simulink model "PLANTA_COMPLETA"  (R2024b)
settings: Solver=FixedStepAuto  StartTime=0.0  StopTime=inf  FixedStep=0.001  MaxStep=0.0005  RelTol=1e-4
undefined symbols (not defined in the file): A_hm, A_tm, at_breakpoints, at_max, b_ha, B_hm, b_ta, B_tm, bcx, bcy, bhd, bhEb, bhm, bt, btd, btm, btw, bwu, C_hm, C_tm, D_hm, D_tm, DiscIntNeverNeededParam, dl_h_ini, dx_l_ini, dx_t_ini, dx_td_ini, dxt_max, dy_l_ini, F01_a_t_max, F01_Ts1, F02_a_h_max, F02_Ts1, F03_a_h_max, F03_a_t_max, F03_dxt_max, F03_Ts1, Fhw_min, g, Hc, ih, it, Jhd_hEb, Jhm_hb, Jtd, Jtm_tb, K_hsa, K_hsia, K_tsa, K_tsia, Kcy, Kd_table, Ke_tita, Ke_w, kp_pos, Kp_table, kp_w, Ktw, kwu, l_breakpoints ... (+30)
libraries: simulink x13, spsEdgeDetectorLib x5, simulink_extras x2, dspsigops x2, vrlib x1, dspstat3 x1
(part 1 of 5)
settings Model: Creator=ribei  LastModifiedBy=juani
settings SolverCC: ZeroCrossAlgorithm=Adaptive  AutoInsertRateTranBlk=on
settings DebuggingCC: IgnoredZcDiagnostic=none  UnderSpecifiedDimensionMsg=warning

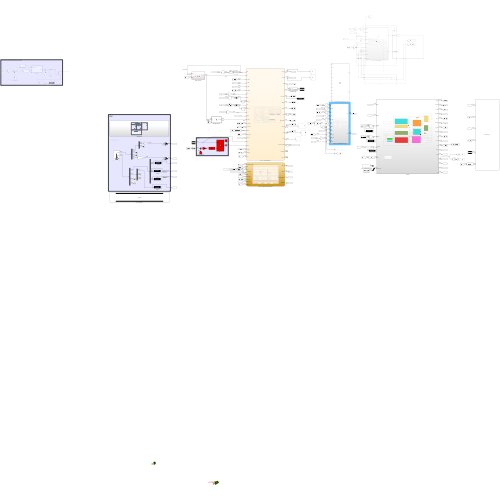
[thumbnail: Simulink's stored preview of the top-level diagram]
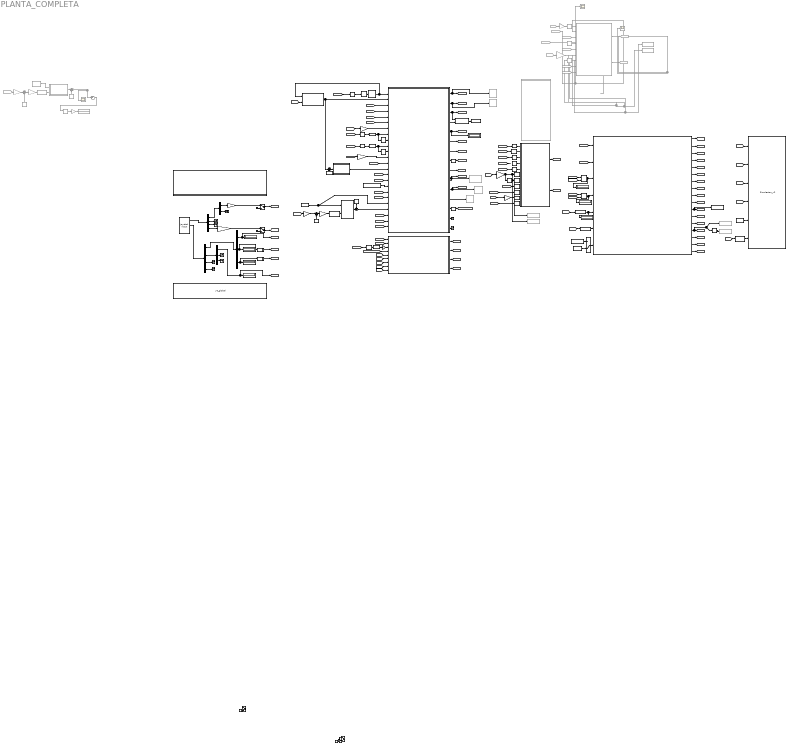
== system PLANTA_COMPLETA ==
  note: SOLO PARA PROBAR ESTIMADOR DE MASA
  note: HMI
  note: LIDAR
  note: CONTROL
  AND : Logic  IconShape=distinctive  AllPortsSameDT=off  OutDataTypeStr=boolean
  AND1 : Logic  IconShape=distinctive  AllPortsSameDT=off  OutDataTypeStr=boolean
  Actualizar perfil : Subsystem
  Ajuste referencia : Constant  Value=30
  Ajuste referencia1 : Constant  Commented=on  Value=30
  Boton A : Display
  Boton B : Display
  Boton X : Display
  Boton Y : Display
  Calculo : MATLAB Function  Commented=on  TreatAsAtomicUnit=on
  Cast : DataTypeConversion  OutDataTypeStr=boolean  SaturateOnIntegerOverflow=off  RndMeth=Floor
  Cast To Boolean : DataTypeConversion  OutDataTypeStr=boolean  SaturateOnIntegerOverflow=off  RndMeth=Floor
  Cast1 : DataTypeConversion  OutDataTypeStr=boolean  SaturateOnIntegerOverflow=off  RndMeth=Floor
  Constant : Constant
  Constant{1..2,18..19,28} (5 alike) : Constant  Value=0  SampleTime=T_s1
  Constant15 : Constant  Value=Yt0
  Constant3 : Constant  Commented=on  Value=Ms
  Constant4 : Constant  Value=30.7948720557058
  Constant5 : Constant  Commented=on
  Constant9 : Constant  Value=Ms
  DASHBOARD : Subsystem
  Data Store Read1 : DataStoreRead  DataStoreName=y0_global  IndexOptions=Index vector (dialog)  Indices=1  OutputSizes=1
  Data Store Read2 : DataStoreRead  DataStoreName=y0_global  IndexOptions=Index vector (dialog)  Indices=1  OutputSizes=1
  Data Store Write : DataStoreWrite  DataStoreName=y0_global  IndexOptions=Index vector (dialog)  Indices=1  OutputSizes=1
  Data Type Conversion : DataTypeConversion  OutDataTypeStr=int32  RndMeth=Ceiling  SaturateOnIntegerOverflow=off
  Data Type Conversion1 : DataTypeConversion  Commented=on  OutDataTypeStr=int32  RndMeth=Ceiling  SaturateOnIntegerOverflow=off
  Delay1 : Delay  DelayLength=1  InputProcessing=Columns as channels (frame based)  SampleTime=T_s1
  Delay2 : Delay  DelayLength=1  InputProcessing=Columns as channels (frame based)  SampleTime=T_s1
  Demux : Demux
  Demux1 : Demux  Outputs=2
  Demux2 : Demux
  Demux3 : Demux  Outputs=3
  Demux4 : Demux  Outputs=3
  Derivative : Derivative  Commented=on
  Derivative1 : Derivative  Commented=on
  Derivative2 : Derivative
  Derivative3 : Derivative
  Discrete Derivative : simulink/Discrete/Discrete Derivative  gainval=1.0  ICPrevScaledInput=0.0  OutMin=[]  OutMax=[]  OutDataType=fixdt(1, 16)  OutScaling=2^-10  DoSatur=off
  Discrete Derivative1 : simulink/Discrete/Discrete Derivative  gainval=1.0  ICPrevScaledInput=0.0  OutMin=[]  OutMax=[]  OutDataType=fixdt(1, 16)  OutScaling=2^-10  DoSatur=off
  Discrete Derivative2 : simulink/Discrete/Discrete Derivative  gainval=1.0  ICPrevScaledInput=0.0  OutMin=[]  OutMax=[]  OutDataType=fixdt(1, 16)  OutScaling=2^-10  DoSatur=off
  Display{,2..4} (4 alike) : Display
  Display1 : Display  Commented=on
  Divide : Product  Commented=on  Inputs=*/
  Enclavamiento : Stateflow chart  TreatAsAtomicUnit=on
  Enclavamiento1 : Stateflow chart  TreatAsAtomicUnit=on
  From1 : From  Commented=on  GotoTag=tita_l
  From11 : From  Commented=on  GotoTag=dxt_ref
  From15 : From  Commented=on  GotoTag=Ml_estimada
  From2 : From  Commented=on  GotoTag=tita_tm
  From21 : From  Commented=on  GotoTag=bal_control
  From22 : From  Commented=on  GotoTag=ddxt_ref
  From3 : From  Commented=on  GotoTag=tita_hm
  From44 : From  Commented=on  GotoTag=dlh_ref
  From5 : From  Commented=on  GotoTag=tita_tm
  Gain : Gain  Gain=1/Wc
  Gain1 : Gain  Commented=on  Gain=rtd/it
  Gain12 : Gain  Gain=rtd/it
  Gain13 : Gain  Gain=-rhd/(ih*2)
  Gain2 : Gain  Commented=on  Gain=-rhd/(ih*2)
  Gain3 : Gain  Gain=rtd/it
  Gain4 : Gain  Gain=rtd/it
  Gain5 : Gain  Gain=-rhd/(ih*2)
  Gain6 : Gain  Commented=on  Gain=1/Wc
  Gain7 : Gain  Commented=on  Gain=rtd/it
  Gain8 : Gain  Gain=rhd/(-2*ih)
  Gain9 : Gain  Commented=on  Gain=100
  Goto10 : Goto  Commented=on  GotoTag=T_tm
  Goto11 : Goto  Commented=on  GotoTag=T_hm
  Joystick Input : vrlib/Joystick Input  joyid=1  adjustports=on  forcefeed=off
  Level-2 MATLAB S-Function : M-S-Function  FunctionName=Simulacion_v2  Parameters=2.438, 2.591, 1.500, 0.850, 0.750, 7.500, 2.100, 2.500, 'black', 'black', '#E99000', 5.000
  Manual Switch{1..4,11} (5 alike) : ManualSwitch
  Manual Switch5 : ManualSwitch  CurrentSetting=0
  Masa contenedor : Subsystem
  Memory1 : Memory  InheritSampleTime=on
  Memory2 : Memory  InheritSampleTime=on
  Moving Average : dspstat3/Moving Average  Method=Sliding window  ForgettingFactorPort=off  SpecifyWindowLength=on  WindowLength=40  OverlapLength=0  AllowArbitraryInputLength=off  ForgettingFactor=0.9  SimulateUsing=Interpreted execution
  Multiply : Gain  Gain=vt_max
  Multiply1 : Gain  Gain=vh_max_sc
  Nivel 0 - Seguridad o Proteccion : Stateflow chart  TreatAsAtomicUnit=on  SystemSampleTime=T_s0
      settings: PortSchema="{\"entries\":[{\"content\":{\"sides\":[{\"content\":{\"connectorIds\":[\"In6\",\"In9\",\"In8\",\"In7\",\"In1\",\"In2\",\"In3\",\"In5\",\"In4\"]},\"type\":\"ConnectorPlacement.EquallySpacedRectSide\",\"uuid\":\"92abb5b4-7f8d-4d16-9e1c-3f1528aec02e\"},{\"content\":{\"connectorIds\":[\"Out2\",\"Out1\",\"Out3\",\"Out4\"],\"side\":\"RIGHT\"},\"type\":\"ConnectorPlacement.EquallySpacedRectSide\",\"uuid\":\"fdfc4918-925b-4492-9924-9f3ed7c6f0ea\"},{\"content\":{\"side\":\"TOP\"},\"type\":\"ConnectorPlacement.EquallySpacedRectSide\",\"uuid\":\"6cd2c614-9727-439b-b51b-96ebe361e1e6\"},{\"content\":{\"side\":\"BOTTOM\"},\"type\":\"ConnectorPlacement.EquallySpacedRectSide\",\"uuid\":\"c327f02f-ffd6-4494-8eea-bb6a75c04a8c\"}]},\"type\":\"ConnectorPlacement.EquallySpacedConnector\",\"uuid\":\"17c891de-27fd-4863-a62e-79c0c94ffbc9\"}],\"packageUris\":[\"http://schema.mathworks.com/mf0/Connector/R2020b\"],\"version\":\"1.0\"}"
  Nivel 1 - Control Supervisor : Stateflow chart  TreatAsAtomicUnit=on  SystemSampleTime=T_s1
  Nivel 2 - Control Regulatorio : Subsystem  Commented=on
  Nivel 2 - Control Regulatorio + Obs : Subsystem
  Nivel 2: Control Regulatorio1 : MATLAB Function  Commented=on  TreatAsAtomicUnit=on  SystemSampleTime=T_s2
  PLANTA : Subsystem
  Perfil de obstaculos : DataStoreMemory  DataStoreName=y0_global  WriteAfterWriteMsg=warning  InitialValue=y0  ShowAdditionalParam=off  OutDataTypeStr=double
  Scope1 : Scope  Commented=on  NumInputPorts=2
  Scope4 : Scope  Commented=on
  Scope5 : Scope  Commented=on
  Sum : Sum  Inputs=|++
  Sum1 : Sum  Inputs=|++
  Sum2 : Sum  Inputs=+-|
  Sum3 : Sum  Commented=on  Inputs=|++
  Sum4 : Sum  Commented=on  Inputs=|++
  Sum5 : Sum  Commented=on  Inputs=-|+||
  Tapped Delay : simulink/Discrete/Tapped Delay  vinit=0.0  samptime=T_s1  NumDelays=40  DelayOrder=Oldest  includeCurrent=off
  Terminator{,1..8} (9 alike) : Terminator
  To Workspace : ToWorkspace  Commented=on  VariableName=xt_ref  SaveFormat=Timeseries  SampleTime=-1
      settings: Save2DSignal=2-D array (concatenate along first dimension)
  To Workspace1 : ToWorkspace  Commented=on  VariableName=ddxt_ref  SaveFormat=Timeseries  SampleTime=-1
      settings: Save2DSignal=2-D array (concatenate along first dimension)
  To Workspace10 : ToWorkspace  Commented=on  VariableName=l_h_real  SaveFormat=Timeseries  SampleTime=-1
      settings: Save2DSignal=2-D array (concatenate along first dimension)
  To Workspace11 : ToWorkspace  Commented=on  VariableName=dl_h_real  SaveFormat=Timeseries  SampleTime=-1
      settings: Save2DSignal=2-D array (concatenate along first dimension)
  To Workspace2 : ToWorkspace  Commented=on  VariableName=dxt_ref  SaveFormat=Timeseries  SampleTime=-1
      settings: Save2DSignal=2-D array (concatenate along first dimension)
  To Workspace3 : ToWorkspace  Commented=on  VariableName=dlh_ref  SaveFormat=Timeseries  SampleTime=-1
      settings: Save2DSignal=2-D array (concatenate along first dimension)
  To Workspace4 : ToWorkspace  Commented=on  VariableName=lh_ref  SaveFormat=Timeseries  SampleTime=-1
      settings: Save2DSignal=2-D array (concatenate along first dimension)
  To Workspace5 : ToWorkspace  Commented=on  VariableName=x_t_real  SaveFormat=Timeseries  SampleTime=-1
      settings: Save2DSignal=2-D array (concatenate along first dimension)
  To Workspace6 : ToWorkspace  Commented=on  VariableName=l_h_real  SaveFormat=Timeseries  SampleTime=-1
      settings: Save2DSignal=2-D array (concatenate along first dimension)
  To Workspace7 : ToWorkspace  Commented=on  VariableName=dl_h_real  SaveFormat=Timeseries  SampleTime=-1
      settings: Save2DSignal=2-D array (concatenate along first dimension)
  To Workspace8 : ToWorkspace  VariableName=tita_real  SaveFormat=Timeseries  SampleTime=-1
      settings: Save2DSignal=2-D array (concatenate along first dimension)
  To Workspace9 : ToWorkspace  Commented=on  VariableName=dx_t_real  SaveFormat=Timeseries  SampleTime=-1
      settings: Save2DSignal=2-D array (concatenate along first dimension)
  Vector de masas : FromWorkspace  VariableName=Mc_Xvect
  Vector de masas sobrecarga : FromWorkspace  VariableName=Mc_Xvect_sobrecarga
  Vector de masas3 : FromWorkspace  Commented=on  VariableName=Mc_Xvect
  Velocidad max izaje : MATLAB Function  TreatAsAtomicUnit=on
  Zero-Order Hold : ZeroOrderHold  SampleTime=T_s1
  Zero-Order Hold1 : ZeroOrderHold  SampleTime=T_s1
  Zero-Order Hold{4..13} (10 alike) : ZeroOrderHold  SampleTime=T_s2
  Zero-Order Hold2 : ZeroOrderHold  SampleTime=T_s1
  Zero-Order Hold3 : ZeroOrderHold  SampleTime=T_s0
  sensor : MATLAB Function  TreatAsAtomicUnit=on
  wires:
  AND/1 -> Display/1, PLANTA/3(BRK_t)
  AND1/1 -> Display3/1, PLANTA/4(BRK_h)
  PLANTA/12(tita_tm) -> [tita_tm]
  PLANTA/13(tita_hm) -> [tita_hm]
  PLANTA/14(x_t) -> Derivative2/1, To Workspace5/1, [x_t]
  PLANTA/15(x_l) -> [x_l]
  PLANTA/16(y_l) -> [y_l]
  Data Store Read2/1 -> Level-2 MATLAB S-Function/5
  [tita_l] -> Level-2 MATLAB S-Function/4
  Gain2/1 -> Nivel 2 - Control Regulatorio/6(l_h), To Workspace10/1, Derivative1/1
  From3/1 -> Gain2/1
  From15/1 -> Nivel 2 - Control Regulatorio/3(m_l)
  Nivel 2 - Control Regulatorio/1(T_tm) -> Scope4/1, Goto10/1
  From2/1 -> Gain1/1  "signal"
  Gain1/1 -> Derivative/1
  Masa contenedor/1(Mc_X) -> Nivel 1 - Control Supervisor/2(Ml), Sum1/1  "signal"
  [FC_SUP] -> Nivel 1 - Control Supervisor/3(FC_SUP)  "signal"
  [FC_INF] -> Nivel 1 - Control Supervisor/4(FC_INF)  "signal"
  [FC_IZQ] -> Nivel 1 - Control Supervisor/5(FC_IZQ)  "signal"
  [FC_DER] -> Nivel 1 - Control Supervisor/6(FC_DER)  "signal"
  Gain3/1 -> Nivel 1 - Control Supervisor/7(xtd)  "signal"
  [tita_hm] -> Zero-Order Hold/1  "signal"
  [tita_tm] -> Zero-Order Hold1/1  "signal"
  Gain5/1 -> Nivel 1 - Control Supervisor/12(lh)  "signal"
  [falla_E] -> Nivel 1 - Control Supervisor/13(falla_E)
  Demux4/1 -> [Boton_A], Boton A/1  "signal"
  Demux4/2 -> Enclavamiento1/1(input), Boton B/1  "signal"
  Constant4/1 -> Nivel 1 - Control Supervisor/17(destino)  "signal"
  Nivel 1 - Control Supervisor/3(TLK) -> [TLK], Actualizar perfil/1(TLK)
  Nivel 1 - Control Supervisor/7(BRK_t) -> [BRK_t_N1]
  Nivel 1 - Control Supervisor/6(BRK_h) -> [BRK_h_N1]
  Nivel 1 - Control Supervisor/5(bal_control) -> [bal_control], Display2/1
  Nivel 1 - Control Supervisor/4(c) -> Actualizar perfil/2(index)
  Nivel 2 - Control Regulatorio/2(T_hm) -> Goto11/1
  [T_tm] -> PLANTA/1(T_tm)
  [T_hm] -> PLANTA/2(T_hm)
  [TLK] -> Cast1/1
  PLANTA/11(tita_l) -> To Workspace8/1, [tita_l]
  [x_t] -> Level-2 MATLAB S-Function/1
  [x_l] -> Level-2 MATLAB S-Function/2
  [y_l] -> Level-2 MATLAB S-Function/3
  PLANTA/1(FC_IZQ) -> [FC_IZQ]
  PLANTA/2(FCE_IZQ) -> [FCE_IZQ]
  PLANTA/3(FC_DER) -> [FC_DER]
  PLANTA/4(FCE_DER) -> [FCE_DER]
  PLANTA/5(FC_INF) -> [FC_INF]
  PLANTA/6(FCE_INF) -> [FCE_INF]
  PLANTA/7(FC_SUP) -> [FC_SUP]
  PLANTA/8(FCE_SUP) -> [FCE_SUP]
  PLANTA/9(Fhw) -> [Fhw]
  PLANTA/10(S_TLK) -> [S_TLK]
  [tita_tm] -> Gain3/1  "signal"
  Discrete Derivative1/1 -> Nivel 1 - Control Supervisor/10(wtm), Delay1/1
  [tita_hm] -> Gain5/1
  Actualizar perfil/1(y0_actualizado) -> Data Store Write/1
  Data Type Conversion/1 -> sensor/2(index)
  Constant15/1 -> Sum2/1
  sensor/1(distancia) -> Sum2/2
  Ajuste referencia/1 -> Sum/2
  Gain4/1 -> Sum/1  "xtd"
  Sum/1 -> Gain/1
  Gain/1 -> Data Type Conversion/1
  [tita_tm] -> Gain4/1  "signal"
  PLANTA/17(Ftw) -> [Ftw]
  Nivel 1 - Control Supervisor/1(dxt_ref) -> To Workspace2/1, [dxt_ref]  "dxt_ref"
  Nivel 1 - Control Supervisor/2(dlh_ref) -> [dlh_ref], To Workspace3/1  "dlh_ref"
  Derivative/1 -> Nivel 2 - Control Regulatorio/1(dx_td)  "dx_td"
  Derivative1/1 -> To Workspace11/1, Nivel 2 - Control Regulatorio/7(dl_h)  "dl_h"
  From11/1 -> Nivel 2 - Control Regulatorio/2(dx_tref), Scope5/1  "dxt_ref"
  From44/1 -> Nivel 2 - Control Regulatorio/5(dl_href)
  Demux/1 -> Demux1/1
  Demux/3 -> Terminator1/1
  Demux1/2 -> Terminator2/1
  Demux/2 -> Terminator/1
  Joystick Input/1 -> Demux/1
  Constant28/1 -> Manual Switch11/2
  ? -> Manual Switch11/1
  Constant1/1 -> Manual Switch1/2
  ? -> Manual Switch1/1
  Constant2/1 -> Manual Switch2/2
  Constant18/1 -> Manual Switch3/2
  Demux1/1 -> Multiply/1  "Carro"
  Constant19/1 -> Manual Switch4/2
  Demux/4 -> Multiply1/1  "Izaje"
  Demux3/1 -> [Boton_Y], Boton Y/1
  Demux3/2 -> Terminator5/1
  Demux4/3 -> Enclavamiento/1(input), Boton X/1
  Demux2/2 -> Demux3/1
  Demux2/4 -> Terminator4/1
  Demux3/3 -> Terminator6/1
  Joystick Input/2 -> Demux2/1
  Demux2/3 -> Terminator3/1
  Demux2/1 -> Demux4/1
  Sum1/1 -> Velocidad max izaje/1(M_l)
  Constant9/1 -> Sum1/2
  [TLK] -> Masa contenedor/2(TLK)
  Velocidad max izaje/1(dxt_max) -> Nivel 1 - Control Supervisor/14(dlh_max)  "signal"
  Multiply1/1 -> Manual Switch4/1
  Discrete Derivative/1 -> Nivel 1 - Control Supervisor/8(whm), Delay2/1
  Delay1/1 -> Nivel 1 - Control Supervisor/11(wtm_ant)
  Zero-Order Hold/1 -> Discrete Derivative/1
  Zero-Order Hold1/1 -> Discrete Derivative1/1
  Sum2/1 -> Nivel 1 - Control Supervisor/21(yc0_xt)
  Data Store Read1/1 -> sensor/1(y0_array), Nivel 1 - Control Supervisor/20(Y_c0)
  [T_tm] -> Nivel 1 - Control Supervisor/22(Ttm_disp)
  [T_hm] -> Nivel 1 - Control Supervisor/23(Thm_disp)
  [Fhw] -> Zero-Order Hold2/1  "signal"
  Moving Average/1 -> Masa contenedor/1(Fwh), Nivel 1 - Control Supervisor/1(Fhw)  "señal filtrada"
  Tapped Delay/1 -> Moving Average/1
  Zero-Order Hold2/1 -> Tapped Delay/1  "señal cruda"
  Vector de masas3/1 -> Calculo/1(masas_array)
  Ajuste referencia1/1 -> Sum3/2
  Sum3/1 -> Gain6/1
  Data Type Conversion1/1 -> Calculo/2(index)
  Gain6/1 -> Data Type Conversion1/1
  From5/1 -> Gain7/1  "signal"
  Gain7/1 -> Sum3/1  "signal"
  Calculo/1(Mc_X) -> Sum4/1
  [TLK] -> Cast To Boolean/1
  Sum4/1 -> Sum5/2, Scope1/2  "Masa real"
  Constant3/1 -> Sum4/2
  Sum5/1 -> Divide/1
  Gain9/1 -> Display1/1
  Divide/1 -> Gain9/1
  Delay2/1 -> Nivel 1 - Control Supervisor/9(whm_ant)
  From1/1 -> Nivel 2 - Control Regulatorio/8(theta)
  Nivel 1 - Control Supervisor/9(Ml_estimada) -> [Ml_estimada]
  From21/1 -> ?
  From22/1 -> Nivel 2 - Control Regulatorio/9(ddx_t_ref)
  Nivel 1 - Control Supervisor/10(ddxt_ref) -> [ddxt_ref], To Workspace1/1  "ddxt_ref"
  Multiply/1 -> Manual Switch3/1
  [tita_l] -> Nivel 1 - Control Supervisor/24(tita_l)
  Manual Switch5/1 -> PLANTA/7(masas_array)
  Vector de masas/1 -> Manual Switch5/2
  Vector de masas sobrecarga/1 -> Manual Switch5/1
  [FCE_IZQ] -> Nivel 0 - Seguridad o Proteccion/3(FCE_IZQ)
  [FCE_DER] -> Nivel 0 - Seguridad o Proteccion/2(FCE_DER)
  [FCE_SUP] -> Nivel 0 - Seguridad o Proteccion/5(FCE_SUP)
  [FCE_INF] -> Nivel 0 - Seguridad o Proteccion/4(FCE_INF)
  Nivel 0 - Seguridad o Proteccion/2(BRK_t) -> [BRK_t_N0]
  Nivel 0 - Seguridad o Proteccion/1(BRK_h) -> [BRK_h_N0]
  Nivel 0 - Seguridad o Proteccion/3(EmergenciaNivel) -> [falla_E]
  [Boton_B] -> Nivel 1 - Control Supervisor/18(balanceo_on)
  [Boton_X] -> Nivel 1 - Control Supervisor/19(TLK_act)
  Enclavamiento1/1(output) -> [Boton_B]  "B"
  Enclavamiento/1(output) -> [Boton_X]  "X"
  [Boton_A] -> Nivel 0 - Seguridad o Proteccion/6(PulsadorEmergecia)
  [Boton_Y] -> Nivel 0 - Seguridad o Proteccion/9(OK)
  Manual Switch4/1 -> [dlh_ref_man]
  Manual Switch3/1 -> [dxt_ref_man]
  [dlh_ref_man] -> Nivel 1 - Control Supervisor/15(dlh_ref_man)
  [dxt_ref_man] -> Nivel 1 - Control Supervisor/16(dxt_ref_man)
  [tita_hm] -> Zero-Order Hold3/1  "signal"
  Zero-Order Hold3/1 -> Discrete Derivative2/1
  Discrete Derivative2/1 -> Gain8/1
  Gain8/1 -> Nivel 0 - Seguridad o Proteccion/8(dlh)
  [alive] -> Nivel 0 - Seguridad o Proteccion/1(alive)
  Nivel 0 - Seguridad o Proteccion/4(BRK_hE) -> [BRK_hE]
  [BRK_t_N0] -> AND/1
  [BRK_t_N1] -> AND/2
  [BRK_h_N0] -> AND1/1
  [BRK_h_N1] -> AND1/2
  Memory1/1 -> [alive]
  Nivel 1 - Control Supervisor/8(alive) -> Memory1/1
  Cast To Boolean/1 -> Level-2 MATLAB S-Function/6
  Nivel 1 - Control Supervisor/13(dlh_max_estimada) -> Memory2/1
  [dlh_max_estimada] -> Nivel 0 - Seguridad o Proteccion/7(v_max_izaje)  "v_max_izaje"
  Memory2/1 -> [dlh_max_estimada]
  Nivel 1 - Control Supervisor/14(sobrecarga) -> Terminator7/1
  Nivel 1 - Control Supervisor/15(op_mode) -> Terminator8/1
  ? -> Sum5/1
  [tita_l] -> Zero-Order Hold10/1
  [Ml_estimada] -> Zero-Order Hold5/1
  [ddxt_ref] -> Zero-Order Hold11/1
  [dxt_ref] -> Zero-Order Hold4/1  "dxt_ref"
  [tita_hm] -> Gain13/1
  [dlh_ref] -> Zero-Order Hold7/1
  [tita_tm] -> Gain12/1  "signal"
  [xt_ref] -> Zero-Order Hold13/1
  Nivel 1 - Control Supervisor/11(xt_ref) -> [xt_ref], To Workspace/1  "xt_ref"
  [Fhw] -> Zero-Order Hold6/1  "signal"
  Derivative2/1 -> To Workspace9/1  "dxt_real"
  Nivel 1 - Control Supervisor/12(lh_ref) -> To Workspace4/1  "lh_ref"
  [bal_control] -> ?
  Constant5/1 -> Nivel 2 - Control Regulatorio/4(BC)
  Zero-Order Hold5/1 -> Nivel 2 - Control Regulatorio + Obs/3(m_l)
  Zero-Order Hold11/1 -> Nivel 2 - Control Regulatorio + Obs/9(ddx_t_ref)
  Zero-Order Hold13/1 -> Nivel 2 - Control Regulatorio + Obs/11(xt_ref)
  Zero-Order Hold4/1 -> Nivel 2 - Control Regulatorio + Obs/2(dx_tref)
  Derivative3/1 -> To Workspace7/1, Zero-Order Hold9/1
  Gain12/1 -> Zero-Order Hold12/1
  Gain13/1 -> To Workspace6/1, Zero-Order Hold8/1, Derivative3/1
  Nivel 2 - Control Regulatorio + Obs/1(T_tm) -> [T_tm]
  Nivel 2 - Control Regulatorio + Obs/2(T_hm) -> [T_hm]
  Zero-Order Hold7/1 -> Nivel 2 - Control Regulatorio + Obs/5(dl_href)
  Zero-Order Hold6/1 -> Nivel 2 - Control Regulatorio + Obs/1(Fhw)
  Zero-Order Hold8/1 -> Nivel 2 - Control Regulatorio + Obs/6(l_h)
  Zero-Order Hold9/1 -> Nivel 2 - Control Regulatorio + Obs/7(dl_h)
  Zero-Order Hold10/1 -> Nivel 2 - Control Regulatorio + Obs/8(theta)
  Zero-Order Hold12/1 -> Nivel 2 - Control Regulatorio + Obs/10(x_td_real)
  [BRK_hE] -> Cast/1
  Cast/1 -> Display4/1, PLANTA/5(BRK_hE)
  Cast1/1 -> PLANTA/6(TLK)
  Constant/1 -> Nivel 2 - Control Regulatorio + Obs/4(BC)

== system PLANTA_COMPLETA/Actualizar perfil ==
  TLK : Inport
  index : Inport  Port=2
  Data Store Read3 : DataStoreRead  DataStoreName=y0_global  IndexOptions=Index vector (dialog)  Indices=1  OutputSizes=1
  Edge Detector1 : spsEdgeDetectorLib/Edge Detector  model=Either  ic=0  Ts=-1
      settings: LibrarySourceBlock=sps_lib/Control/Edge Detector
  Enabled Subsystem : Subsystem  TreatAsAtomicUnit=on
  Switch : Switch  Criteria=u2 > Threshold  SaturateOnIntegerOverflow=off  InputSameDT=off
  Unit Delay : UnitDelay  SampleTime=-1  HasFrameUpgradeWarning=on
  y0_actualizado : Outport
  wires:
  Unit Delay/1 -> Edge Detector1/1
  TLK/1 -> Unit Delay/1
  Edge Detector1/1 -> Switch/2, Enabled Subsystem/Enable
  Enabled Subsystem/1(y0_actualizado) -> Switch/1
  index/1 -> Enabled Subsystem/1(index)
  Switch/1 -> y0_actualizado/1
  Data Store Read3/1 -> Switch/3
